simulink model "pidexemplo1"  (R2018a)
settings: Solver=FixedStepAuto  StartTime=0.0  StopTime=2  FixedStep=0.002  RelTol=1e-3
model workspace (MAT data in the model file):
  G1 = tf
  G1.IOSize_ = [2 1]
  G1.Data_ = ltipack.tfdata
  G1.Data_.num = {[0 0 257.593143339 3.66061873562e-12 -14343.2545723]; [0 0 -1762.15858752 -22276.163509]}
  G1.Data_.den = {[1 324.977040995 102.612494515 -17929.0682153 0]; [1 324.977040995 102.612494515 -17929.0682153]}
  G1.Data_.Delay.Input = 0
  G1.Data_.Delay.Output = [0; 0]
  G1.Data_.Delay.IO = [0; 0]
  G1.Data_.Ts = 0
values from neighbouring files (symbols this model uses):
  b = 0.002    [roboteste2.m]
  den = [A B C D]    [roboteste2.m]
  kd = 15.3942    [roboteste2.m]
  ki = 0.0215    [roboteste2.m]
  kp = 39.4946    [roboteste2.m]
  num = [mp*L/q 0]    [roboteste2.m]
undefined symbols (not defined in the file or in its folder): a, c, d
libraries: simulink x4, sh_lib x1, checkpacklib x1, cstblocks x1
settings Model: Creator=Pedro  LastModifiedBy=Pedro
settings SolverCC: PositivePriorityOrder=on

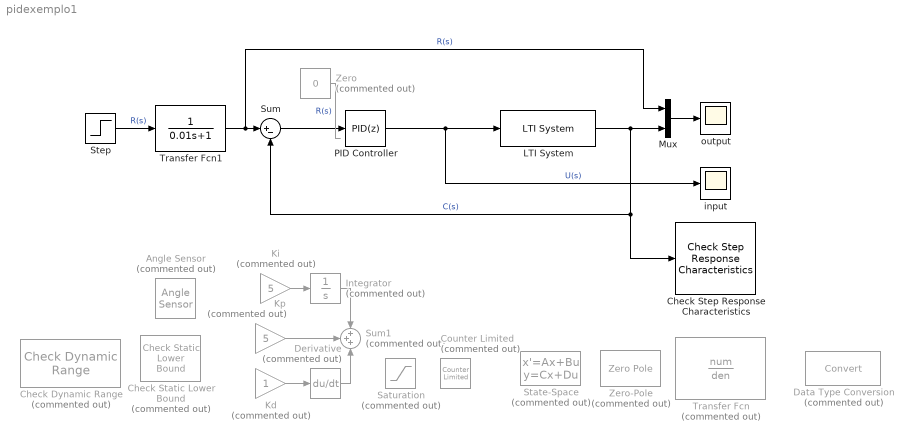
== system pidexemplo1 ==
  Angle Sensor : sh_lib/Pumps and Motors/Angle Sensor  Commented=on  phase_angle=0 deg
      settings: SourceProductName=Simscape Fluids  SourceProductBaseCode=SH
  Check Dynamic Range : simulink/Model Verification/Check  Dynamic Range  Description=min < u < max  Commented=on  enabled=on  stopWhenAssertionFail=on  export=off  icon=graphic
      settings: SourceProductName=Simulink  SourceProductBaseCode=SL
  Check Static Lower Bound : simulink/Model Verification/Check Static  Lower Bound  Description=0 <= u  Commented=on  min=0  min_included=on  enabled=on  stopWhenAssertionFail=on  export=off  icon=graphic
      settings: SourceProductName=Simulink
  Check Step Response Characteristics : checkpacklib/Check Step Response  Characteristics  InstantiateOnLoad=on  enabled=on  stopWhenAssertionFail=off  export=off  ViewDlgPos=[100 200 510 390]  OpenViewOnLoad=on  LaunchViewOnOpen=on  TimeUnits=seconds  EnableStepResponseBound=on  InitialValue=0  FinalValue=1  StepTime=0.002  RiseTime=2  PercentRise=80  SettlingTime=3  PercentSettling=1  PercentOvershoot=10  PercentUndershoot=1
  Counter Limited : simulink/Sources/Counter Limited  Commented=on  uplimit=7  tsamp=-1
  Data Type Conversion : DataTypeConversion  Commented=on
  Derivative : Derivative  Commented=on
  Integrator : Integrator  Commented=on
  Kd : Gain  Commented=on
  Ki : Gain  Commented=on  Gain=5
  Kp : Gain  Commented=on  Gain=5
  LTI System : cstblocks/LTI System  sys=H  IC=[]
  Mux : Mux  Inputs=2
  PID Controller : simulink/Continuous/PID Controller  Controller=PID  TimeDomain=Discrete-time  SampleTime=-1  IntegratorMethod=Forward Euler  FilterMethod=Forward Euler  Form=Parallel  UseFilter=off  ControllerParametersSource=internal  P=kp  I=ki  D=kd  N=2359.46899179402  InitialConditionSource=internal  InitialConditionForIntegrator=0  InitialConditionForFilter=0  ExternalReset=none  LimitOutput=off  UpperSaturationLimit=2  LowerSaturationLimit=-2  LinearizeAsGain=off  AntiWindupMode=none  Kb=1  TrackingMode=off  Kt=1  PParamMin=[]  PParamMax=[]  IParamMin=[]  IParamMax=[]  DParamMin=[]  DParamMax=[]  NParamMin=[]  NParamMax=[]  KbParamMin=[]  KbParamMax=[]  KtParamMin=[]  KtParamMax=[]  POutMin=[]  POutMax=[]  IOutMin=[]  IOutMax=[]  DOutMin=[]  DOutMax=[]  NOutMin=[]  NOutMax=[]  KbOutMin=[]  KbOutMax=[]  KtOutMin=[]  KtOutMax=[]  IntegratorOutMin=[]  IntegratorOutMax=[]  FilterOutMin=[]  FilterOutMax=[]  SumOutMin=[]  SumOutMax=[]  SumI1OutMin=[]  SumI1OutMax=[]  SumI2OutMin=[]  SumI2OutMax=[]  SumI3OutMin=[]  SumI3OutMax=[]  SumDOutMin=[]  SumDOutMax=[]  SaturationOutMin=[]  SaturationOutMax=[]  IntegratorContinuousStateAttributes=''  IntegratorStateMustResolveToSignalObject=off  IntegratorRTWStateStorageClass=Auto  FilterContinuousStateAttributes=''  FilterStateMustResolveToSignalObject=off  FilterRTWStateStorageClass=Auto  DifferentiatorICPrevScaledInput=0  DifferentiatorOutMin=[]  DifferentiatorOutMax=[]  FilterDiffOutCoefMin=[]  FilterDiffOutCoefMax=[]  SumDenOutMin=[]  SumDenOutMax=[]  SumNumOutMin=[]  SumNumOutMax=[]  ReciprocalOutMin=[]  ReciprocalOutMax=[]  DivideOutMin=[]  DivideOutMax=[]  TunerSelectOption=Transfer Function Based (PID Tuner App)
  Saturation : Saturate  Commented=on  UpperLimit=7  LowerLimit=-7
  State-Space : StateSpace  Commented=on  A=a  B=b  C=c  D=d  InitialCondition=0
  Step : Step  Time=0.5  SampleTime=0.0
  Sum : Sum  Inputs=|+-
  Sum1 : Sum  Commented=on  Inputs=+++
  Transfer Fcn : TransferFcn  Commented=on  Numerator=num  Denominator=den
  Transfer Fcn1 : TransferFcn  Denominator=[0.01,1]
  Zero : Constant  Commented=on  Value=0
  Zero-Pole : ZeroPole  Commented=on  Poles=[0 -1]
  input : Scope
  output : Scope
  wires:
  LTI System/1 -> Mux/2, Check Step Response Characteristics/1, Sum/2  "C(s)"
  Mux/1 -> output/1
  PID Controller/1 -> input/1, LTI System/1  "U(s)"
  Step/1 -> Transfer Fcn1/1  "R(s)"
  Derivative/1 -> Sum1/3
  Ki/1 -> Integrator/1
  Kp/1 -> Sum1/2
  Kd/1 -> Derivative/1
  Integrator/1 -> Sum1/1
  Sum/1 -> PID Controller/1
  Zero/1 -> ?  "R(s)"
  Transfer Fcn1/1 -> Mux/1, Sum/1  "R(s)"
